simulink model "Quadcopter_State_model_Arduino"  (R2023b)
settings: Solver=VariableStepAuto  StartTime=0.0  StopTime=inf  FixedStep=0.00001  MinStep=0.001  RelTol=1e-3
model workspace (MAT data in the model file):
  DesiredPitchRoll : sugfis (value not decoded)
  DesiredThrust : sugfis (value not decoded)
  DesiredYaw : sugfis (value not decoded)
  Desired_Pitch = 0
  Desired_Roll = 0
  Desired_Yaw = 0
  Desired_Z_Velocity = -3
  FuzzyMotorspeed : sugfis (value not decoded)
values from neighbouring files (symbols this model uses):
  g = 9.81    [Quadcopter_Constants.m]
  Ixx = 0.0294838    [Quadcopter_Constants.m]
  Iyy = 0.0294838    [Quadcopter_Constants.m]
  Izz = 0.058967624    [Quadcopter_Constants.m]
  Jr = (6e-5)*1.358    (= 8.148e-05)    [Quadcopter_Constants.m]
  kd = 1    [Quadcopter_Constants.m]
  kd_phi = 1    [Quadcopter_Constants.m]
  kd_theta = 1    [Quadcopter_Constants.m]
  kf = 1    [Quadcopter_Constants.m]
  ki = 1    [Quadcopter_Constants.m]
  ki_phi = 1    [Quadcopter_Constants.m]
  ki_theta = 1    [Quadcopter_Constants.m]
  km = 4.74157e-9    (= 4.74157e-09)    [Quadcopter_Constants.m]
  kp = 1    [Quadcopter_Constants.m]
  kp_phi = 1    [Quadcopter_Constants.m]
  kp_theta = 1    [Quadcopter_Constants.m]
  kr = (0.1)*1.358    (= 0.1358)    [Quadcopter_Constants.m]
  kt = (0.1)*1.358    (= 0.1358)    [Quadcopter_Constants.m]
  l = 0.254    [Quadcopter_Constants.m]
  m = 0.914    [Quadcopter_Constants.m]
  sample_freq = 1000    [Quadcopter_Constants.m]
undefined symbols (not defined in the file or in its folder): LF
libraries: fuzblock x18, instrumentseriallib x12, simulink_extras x6, vrlib x4, instrumentlib x3, etargetslib x1, slpidlib x1, simulink x1
(part 2 of 5)

== system Quadcopter_State_model_Arduino/Arduino Sim/Control Panel ==
  note: Control Panel
  note: Enabling Results in
      | Simulation Lag
  Rocker Switch : RockerSwitchBlock
      settings: Values={{'Off', 'On'}, [0 1]}
  Rocker Switch1 : RockerSwitchBlock
      settings: Values={{'Off', 'On'}, [0 1]}
  Rocker Switch2 : RockerSwitchBlock
      settings: Values={{'Off', 'On'}, [0 1]}
  Rotary Switch : CustomTuningWebBlock  LabelPosition=Bottom  ShowInitialText=on  Configuration="{\"components\":[{\"name\":\"RotarySwitchComponent\",\"settings\":{\"arcAngle\":300,\"arcAngleOffset\":120,\"handle\":{\"size\":[150,150],\"src\":\"data:image\\/svg+xml;base64,PHN2ZyBpZD0iTGF5ZXJfMSIgZGF0YS1uYW1lPSJMYXllciAxIiB4bWxucz0iaHR0cDovL3d3dy53My5vcmcvMjAwMC9zdmciIHhtbG5zOnhsaW5rPSJodHRwOi8vd3d3LnczLm9yZy8xOTk5L3hsaW5rIiB2aWV3Qm94PSIwIDAgMTIxIDEyMSI+PGRlZnM+PHN0eWxlPi5jbHMtMXtmaWxsOnVybCgjbGluZWFyLWdyYWRpZW50KTt9LmNscy0yLC5jbHMtM3tmaWxsOiNkMWQxZDE7fS5jbHMtM3tzdHJva2U6I2I3YjdiNztzdHJva2UtbWl0ZXJsaW1pdDoxMDtzdHJva2Utd2lkdGg6MC4yNXB4O30uY2xzLTR7ZmlsbDojZjMwMDAwO30uY2xzLTV7ZmlsbDojZjIxNzY3O308L3N0eWxlPjxsaW5lYXJHcmFkaWVudCBpZD0ibGluZWFyLWdyYWRpZW50IiB4MT0iNjAuNSIgeTE9IjEyMC41IiB4Mj0iNjAuNSIgeTI9IjAuNSIgZ3JhZGllbnRVbml0cz0idXNlclNwYWNlT25Vc2UiPjxzdG9wIG9mZnNldD0iMCIgc3RvcC1jb2xvcj0iI2QxZDFkMSIvPjxzdG9wIG9mZnNldD0iMC4xIiBzdG9wLWNvbG9yPSIjY2VjZWNlIi8+PHN0b3Agb2Zmc2V0PSIwLjE5IiBzdG9wLWNvbG9yPSIjYzNjM2MzIi8+PHN0b3Agb2Zmc2V0PSIwLjI4IiBzdG9wLWNvbG9yPSIjYjFiMWIxIi8+PHN0b3Agb2Zmc2V0PSIwLjM2IiBzdG9wLWNvbG9yPSIjOTg5ODk4Ii8+PHN0b3Agb2Zmc2V0PSIwLjQ0IiBzdG9wLWNvbG9yPSIjNzg3ODc4Ii8+PHN0b3Agb2Zmc2V0PSIwLjQ2IiBzdG9wLWNvbG9yPSIjNmI2YjZiIi8+PHN0b3Agb2Zmc2V0PSIwLjU0IiBzdG9wLWNvbG9yPSIjNmI2YjZiIi8+PHN0b3Agb2Zmc2V0PSIwLjU2IiBzdG9wLWNvbG9yPSIjNzY3Njc2Ii8+PHN0b3Agb2Zmc2V0PSIwLjY0IiBzdG9wLWNvbG9yPSIjOTc5Nzk3Ii8+PHN0b3Agb2Zmc2V0PSIwLjcyIiBzdG9wLWNvbG9yPSIjYjBiMGIwIi8+PHN0b3Agb2Zmc2V0PSIwLjgxIiBzdG9wLWNvbG9yPSIjYzNjM2MzIi8+PHN0b3Agb2Zmc2V0PSIwLjkiIHN0b3AtY29sb3I9IiNjZGNkY2QiLz48c3RvcCBvZmZzZXQ9IjEiIHN0b3AtY29sb3I9IiNkMWQxZDEiLz48L2xpbmVhckdyYWRpZW50PjwvZGVmcz48Y2lyY2xlIGNsYXNzPSJjbHMtMSIgY3g9IjYwLjUiIGN5PSI2MC41IiByPSI2MCIvPjxwYXRoIGNsYXNzPSJjbHMtMiIgZD0iTTYwLjUsMUE1OS41LDU5LjUsMCwxLDEsMSw2MC41LDU5LjU3LDU5LjU3LDAsMCwxLDYwLjUsMW0wLTFBNjAuNSw2MC41LDAsMSwwLDEyMSw2MC41LDYwLjUsNjAuNSwwLDAsMCw2MC41LDBaIi8+PHJlY3QgY2xhc3M9ImNscy0zIiB4PSIwLjUiIHk9IjUxLjUiIHdpZHRoPSIxMjAiIGhlaWdodD0iMTgiIHJ4PSIzLjA0Ii8+PHJlY3QgY2xhc3M9ImNscy00IiB4PSI1Ljc1IiB5PSI1OC43NSIgd2lkdGg9IjE2IiBoZWlnaHQ9IjMiLz48cGF0aCBjbGFzcz0iY2xzLTUiIGQ9Ik0yMS4yNSw1OS4yNXYyaC0xNXYtMmgxNW0xLTFoLTE3djRoMTd2LTRaIi8+PC9zdmc+\"},\"handleOffset\":[0,0],\"handleOrientation\":180,\"handlePosition\":[0,0,1,1],\"handleSize\":{\"height\":0.5,\"width\":0.5},\"labelRadius\":0.36,\"position\":[0,0,1,1],\"states\":[{\"Label\":{\"color\":[0,0,0,1],\"icon\":{\"size\":[0,0],\"src\":[],\"srcOrientation\":\"Right\"},\"iconPlacement\":\"left\",\"opacity\":1,\"position\":[0.7345552884615385,0.6796274038461538],\"show\":true,\"text\":{\"content\":\"-128\",\"font\":\"Helvetica\",\"fontSize\":24}},\"Value\":-128},{\"Label\":{\"color\":[0,0,0,1],\"icon\":{\"size\":[0,0],\"src\":[],\"srcOrientation\":\"Right\"},\"iconPlacement\":\"left\",\"opacity\":1,\"position\":[0.36532451923076925,0.1180889423076923],\"show\":true,\"text\":{\"content\":\"-97\",\"font\":\"Helvetica\",\"fontSize\":24}},\"Value\":-97},{\"Label\":{\"color\":[0,0,0,1],\"icon\":{\"size\":[0,0],\"src\":[],\"srcOrientation\":\"Right\"},\"iconPlacement\":\"left\",\"opacity\":1,\"position\":[0.7191706730769231,0.19501201923076922],\"show\":true,\"text\":{\"content\":\"-65\",\"font\":\"Helvetica\",\"fontSize\":24}},\"Value\":-65},{\"Label\":{\"color\":[0,0,0,1],\"icon\":{\"size\":[0,0],\"src\":[],\"srcOrientation\":\"Right\"},\"iconPlacement\":\"left\",\"opacity\":1,\"position\":[0.35757211538461536,0.7603966346153846],\"show\":true,\"text\":{\"content\":\"-33\",\"font\":\"Helvetica\",\"fontSize\":24}},\"Value\":-33},{\"Label\":{\"color\":[0,0,0,1],\"icon\":{\"size\":[0,0],\"src\":[],\"srcOrientation\":\"Right\"},\"iconPlacement\":\"left\",\"opacity\":1,\"position\":[0.09603365384615385,0.46033653846153844],\"show\":true,\"text\":{\"content\":\"0\",\"font\":\"Helvetica\",\"fontSize\":24}},\"Value\":0},{\"Label\":{\"color\":[0,0,0,1],\"icon\":{\"size\":[0,0],\"src\":[],\"srcOrientation\":\"Right\"},\"iconPlacement\":\"left\",\"opacity\":1,\"position\":[0.7191706730769231,0.19501201923076922],\"show\":true,\"text\":{\"content\":\"32\",\"font\":\"Helvetica\",\"fontSize\":24}},\"Value\":32},{\"Label\":{\"color\":[0,0,0,1],\"icon\":{\"size\":[0,0],\"src\":[],\"srcOrientation\":\"Right\"},\"iconPlacement\":\"left\",\"opacity\":1,\"position\":[0.7191706730769231,0.19501201923076922],\"show\":true,\"text\":{\"content\":\"64\",\"font\":\"Helvetica\",\"fontSize\":24}},\"Value\":64},{\"Label\":{\"color\":[0,0,0,1],\"icon\":{\"size\":[0,0],\"src\":[],\"srcOrientation\":\"Right\"},\"iconPlacement\":\"left\",\"opacity\":1,\"position\":[0.7191706730769231,0.19501201923076922],\"show\":true,\"text\":{\"content\":\"96\",\"font\":\"Helvetica\",\"fontSize\":24}},\"Value\":96},{\"Label\":{\"color\":[0,0,0,1],\"icon\":{\"size\":[0,0],\"src\":[],\"srcOrientation\":\"Right\"},\"iconPlacement\":\"left\",\"opacity\":1,\"position\":[0.7191706730769231,0.19501201923076922],\"show\":true,\"text\":{\"content\":\"127\",\"font\":\"Helvetica\",\"fontSize\":24}},\"Value\":127}],\"tickRadius\":0.32}},{\"name\":\"BackgroundImageComponent\",\"settings\":{\"image\":{\"size\":[155,150],\"src\":\"data:image\\/svg+xml;base64,PD94bWwgdmVyc2lvbj0iMS4wIiBlbmNvZGluZz0idXRmLTgiPz4NCjwhLS0gR2VuZXJhdG9yOiBBZG9iZSBJbGx1c3RyYXRvciAyNS4wLjAsIFNWRyBFeHBvcnQgUGx1Zy1JbiAuIFNWRyBWZXJzaW9uOiA2LjAwIEJ1aWxkIDApICAtLT4NCjxzdmcgdmVyc2lvbj0iMS4xIg0KCSBpZD0iTGF5ZXJfMl8xXyIgeG1sbnM6Y2M9Imh0dHA6Ly9jcmVhdGl2ZWNvbW1vbnMub3JnL25zIyIgeG1sbnM6ZGM9Imh0dHA6Ly9wdXJsLm9yZy9kYy9lbGVtZW50cy8xLjEvIiB4bWxuczppbmtzY2FwZT0iaHR0cDovL3d3dy5pbmtzY2FwZS5vcmcv ...(+4184 chars)\",\"srcOrientation\":\"Right\"},\"position\":[0,0,1,1],\"scaleMode\":\"0\"}},{\"name\":\"ForegroundImageComponent\",\"settings\":{\"image\":{\"size\":[0,0],\"src\":\"default\",\"srcOrientation\":[]},\"isForeground\":1,\"position\":[0,0,1,1],\"scaleMode\":\"0\"}}],\"settings\":{\"BindingType\":\"param\",\"backgroundColor\":[0,0,255,\"1\"],\"backgroundOffset\":1,\"fixedAspectRatio\":\"on\",\"image\":{\"size\":[150,150],\"src\":\"data:image\\/svg+xml;base64,PD94bWwgdmVyc2lvbj0iMS4wIiBlbmNvZGluZz0iVVRGLTgiIHN0YW5kYWxvbmU9Im5vIj8+CjwhLS0gR2VuZXJhdG9yOiBBZG9iZSBJbGx1c3RyYXRvciAxOS4yLjEsIFNWRyBFeHBvcnQgUGx1Zy1JbiAuIFNWRyBWZXJzaW9uOiA2LjAwIEJ1aWxkIDApICAtLT4KCjxzdmcKICAgeG1sbnM6ZGM9Imh0dHA6Ly9wdXJsLm9yZy9kYy9lbGVtZW50cy8xLjEvIgogICB4bWxuczpjYz0iaHR0cDovL2NyZWF0aXZlY29tbW9ucy5vcmcvbnMjIgogICB4bWxuczpyZGY9Imh0dHA6Ly93d3cudzMub3JnLzE5OTkvMDIvMjItcmRmLXN5bnRh ...(+9660 chars)\"},\"showBackgroundColor\":false,\"variant\":\"rotarySwitch\",\"version\":\"R2022b\"},\"type\":\"RotarySwitch\"}"
  Rotary Switch1 : CustomTuningWebBlock  LabelPosition=Bottom  ShowInitialText=on  Configuration="{\"components\":[{\"name\":\"RotarySwitchComponent\",\"settings\":{\"arcAngle\":300,\"arcAngleOffset\":120,\"handle\":{\"size\":[150,150],\"src\":\"data:image\\/svg+xml;base64,PHN2ZyBpZD0iTGF5ZXJfMSIgZGF0YS1uYW1lPSJMYXllciAxIiB4bWxucz0iaHR0cDovL3d3dy53My5vcmcvMjAwMC9zdmciIHhtbG5zOnhsaW5rPSJodHRwOi8vd3d3LnczLm9yZy8xOTk5L3hsaW5rIiB2aWV3Qm94PSIwIDAgMTIxIDEyMSI+PGRlZnM+PHN0eWxlPi5jbHMtMXtmaWxsOnVybCgjbGluZWFyLWdyYWRpZW50KTt9LmNscy0yLC5jbHMtM3tmaWxsOiNkMWQxZDE7fS5jbHMtM3tzdHJva2U6I2I3YjdiNztzdHJva2UtbWl0ZXJsaW1pdDoxMDtzdHJva2Utd2lkdGg6MC4yNXB4O30uY2xzLTR7ZmlsbDojZjMwMDAwO30uY2xzLTV7ZmlsbDojZjIxNzY3O308L3N0eWxlPjxsaW5lYXJHcmFkaWVudCBpZD0ibGluZWFyLWdyYWRpZW50IiB4MT0iNjAuNSIgeTE9IjEyMC41IiB4Mj0iNjAuNSIgeTI9IjAuNSIgZ3JhZGllbnRVbml0cz0idXNlclNwYWNlT25Vc2UiPjxzdG9wIG9mZnNldD0iMCIgc3RvcC1jb2xvcj0iI2QxZDFkMSIvPjxzdG9wIG9mZnNldD0iMC4xIiBzdG9wLWNvbG9yPSIjY2VjZWNlIi8+PHN0b3Agb2Zmc2V0PSIwLjE5IiBzdG9wLWNvbG9yPSIjYzNjM2MzIi8+PHN0b3Agb2Zmc2V0PSIwLjI4IiBzdG9wLWNvbG9yPSIjYjFiMWIxIi8+PHN0b3Agb2Zmc2V0PSIwLjM2IiBzdG9wLWNvbG9yPSIjOTg5ODk4Ii8+PHN0b3Agb2Zmc2V0PSIwLjQ0IiBzdG9wLWNvbG9yPSIjNzg3ODc4Ii8+PHN0b3Agb2Zmc2V0PSIwLjQ2IiBzdG9wLWNvbG9yPSIjNmI2YjZiIi8+PHN0b3Agb2Zmc2V0PSIwLjU0IiBzdG9wLWNvbG9yPSIjNmI2YjZiIi8+PHN0b3Agb2Zmc2V0PSIwLjU2IiBzdG9wLWNvbG9yPSIjNzY3Njc2Ii8+PHN0b3Agb2Zmc2V0PSIwLjY0IiBzdG9wLWNvbG9yPSIjOTc5Nzk3Ii8+PHN0b3Agb2Zmc2V0PSIwLjcyIiBzdG9wLWNvbG9yPSIjYjBiMGIwIi8+PHN0b3Agb2Zmc2V0PSIwLjgxIiBzdG9wLWNvbG9yPSIjYzNjM2MzIi8+PHN0b3Agb2Zmc2V0PSIwLjkiIHN0b3AtY29sb3I9IiNjZGNkY2QiLz48c3RvcCBvZmZzZXQ9IjEiIHN0b3AtY29sb3I9IiNkMWQxZDEiLz48L2xpbmVhckdyYWRpZW50PjwvZGVmcz48Y2lyY2xlIGNsYXNzPSJjbHMtMSIgY3g9IjYwLjUiIGN5PSI2MC41IiByPSI2MCIvPjxwYXRoIGNsYXNzPSJjbHMtMiIgZD0iTTYwLjUsMUE1OS41LDU5LjUsMCwxLDEsMSw2MC41LDU5LjU3LDU5LjU3LDAsMCwxLDYwLjUsMW0wLTFBNjAuNSw2MC41LDAsMSwwLDEyMSw2MC41LDYwLjUsNjAuNSwwLDAsMCw2MC41LDBaIi8+PHJlY3QgY2xhc3M9ImNscy0zIiB4PSIwLjUiIHk9IjUxLjUiIHdpZHRoPSIxMjAiIGhlaWdodD0iMTgiIHJ4PSIzLjA0Ii8+PHJlY3QgY2xhc3M9ImNscy00IiB4PSI1Ljc1IiB5PSI1OC43NSIgd2lkdGg9IjE2IiBoZWlnaHQ9IjMiLz48cGF0aCBjbGFzcz0iY2xzLTUiIGQ9Ik0yMS4yNSw1OS4yNXYyaC0xNXYtMmgxNW0xLTFoLTE3djRoMTd2LTRaIi8+PC9zdmc+\"},\"handleOffset\":[0,0],\"handleOrientation\":180,\"handlePosition\":[0,0,1,1],\"handleSize\":{\"height\":0.5,\"width\":0.5},\"labelRadius\":0.36,\"position\":[0,0,1,1],\"states\":[{\"Label\":{\"color\":[0,0,0,1],\"icon\":{\"size\":[0,0],\"src\":[],\"srcOrientation\":\"Right\"},\"iconPlacement\":\"left\",\"opacity\":1,\"position\":[0.7345552884615385,0.6796274038461538],\"show\":true,\"text\":{\"content\":\"-127\",\"font\":\"Helvetica\",\"fontSize\":24}},\"Value\":-127},{\"Label\":{\"color\":[0,0,0,1],\"icon\":{\"size\":[0,0],\"src\":[],\"srcOrientation\":\"Right\"},\"iconPlacement\":\"left\",\"opacity\":1,\"position\":[0.36532451923076925,0.1180889423076923],\"show\":true,\"text\":{\"content\":\"-96\",\"font\":\"Helvetica\",\"fontSize\":24}},\"Value\":-96},{\"Label\":{\"color\":[0,0,0,1],\"icon\":{\"size\":[0,0],\"src\":[],\"srcOrientation\":\"Right\"},\"iconPlacement\":\"left\",\"opacity\":1,\"position\":[0.7191706730769231,0.19501201923076922],\"show\":true,\"text\":{\"content\":\"-64\",\"font\":\"Helvetica\",\"fontSize\":24}},\"Value\":-64},{\"Label\":{\"color\":[0,0,0,1],\"icon\":{\"size\":[0,0],\"src\":[],\"srcOrientation\":\"Right\"},\"iconPlacement\":\"left\",\"opacity\":1,\"position\":[0.35757211538461536,0.7603966346153846],\"show\":true,\"text\":{\"content\":\"-32\",\"font\":\"Helvetica\",\"fontSize\":24}},\"Value\":-32},{\"Label\":{\"color\":[0,0,0,1],\"icon\":{\"size\":[0,0],\"src\":[],\"srcOrientation\":\"Right\"},\"iconPlacement\":\"left\",\"opacity\":1,\"position\":[0.09603365384615385,0.46033653846153844],\"show\":true,\"text\":{\"content\":\"0\",\"font\":\"Helvetica\",\"fontSize\":24}},\"Value\":0},{\"Label\":{\"color\":[0,0,0,1],\"icon\":{\"size\":[0,0],\"src\":[],\"srcOrientation\":\"Right\"},\"iconPlacement\":\"left\",\"opacity\":1,\"position\":[0.7191706730769231,0.19501201923076922],\"show\":true,\"text\":{\"content\":\"32\",\"font\":\"Helvetica\",\"fontSize\":24}},\"Value\":32},{\"Label\":{\"color\":[0,0,0,1],\"icon\":{\"size\":[0,0],\"src\":[],\"srcOrientation\":\"Right\"},\"iconPlacement\":\"left\",\"opacity\":1,\"position\":[0.7191706730769231,0.19501201923076922],\"show\":true,\"text\":{\"content\":\"64\",\"font\":\"Helvetica\",\"fontSize\":24}},\"Value\":64},{\"Label\":{\"color\":[0,0,0,1],\"icon\":{\"size\":[0,0],\"src\":[],\"srcOrientation\":\"Right\"},\"iconPlacement\":\"left\",\"opacity\":1,\"position\":[0.7191706730769231,0.19501201923076922],\"show\":true,\"text\":{\"content\":\"96\",\"font\":\"Helvetica\",\"fontSize\":24}},\"Value\":96},{\"Label\":{\"color\":[0,0,0,1],\"icon\":{\"size\":[0,0],\"src\":[],\"srcOrientation\":\"Right\"},\"iconPlacement\":\"left\",\"opacity\":1,\"position\":[0.7191706730769231,0.19501201923076922],\"show\":true,\"text\":{\"content\":\"127\",\"font\":\"Helvetica\",\"fontSize\":24}},\"Value\":127}],\"tickRadius\":0.32}},{\"name\":\"BackgroundImageComponent\",\"settings\":{\"image\":{\"size\":[155,150],\"src\":\"data:image\\/svg+xml;base64,PD94bWwgdmVyc2lvbj0iMS4wIiBlbmNvZGluZz0idXRmLTgiPz4NCjwhLS0gR2VuZXJhdG9yOiBBZG9iZSBJbGx1c3RyYXRvciAyNS4wLjAsIFNWRyBFeHBvcnQgUGx1Zy1JbiAuIFNWRyBWZXJzaW9uOiA2LjAwIEJ1aWxkIDApICAtLT4NCjxzdmcgdmVyc2lvbj0iMS4xIg0KCSBpZD0iTGF5ZXJfMl8xXyIgeG1sbnM6Y2M9Imh0dHA6Ly9jcmVhdGl2ZWNvbW1vbnMub3JnL25zIyIgeG1sbnM6ZGM9Imh0dHA6Ly9wdXJsLm9yZy9kYy9lbGVtZW50cy8xLjEvIiB4bWxuczppbmtzY2FwZT0iaHR0cDovL3d3dy5pbmtzY2FwZS5vcmcv ...(+4184 chars)\",\"srcOrientation\":\"Right\"},\"position\":[0,0,1,1],\"scaleMode\":\"0\"}},{\"name\":\"ForegroundImageComponent\",\"settings\":{\"image\":{\"size\":[0,0],\"src\":\"default\",\"srcOrientation\":[]},\"isForeground\":1,\"position\":[0,0,1,1],\"scaleMode\":\"0\"}}],\"settings\":{\"BindingType\":\"param\",\"backgroundColor\":[0,0,255,\"1\"],\"backgroundOffset\":1,\"fixedAspectRatio\":\"on\",\"image\":{\"size\":[150,150],\"src\":\"data:image\\/svg+xml;base64,PD94bWwgdmVyc2lvbj0iMS4wIiBlbmNvZGluZz0iVVRGLTgiIHN0YW5kYWxvbmU9Im5vIj8+CjwhLS0gR2VuZXJhdG9yOiBBZG9iZSBJbGx1c3RyYXRvciAxOS4yLjEsIFNWRyBFeHBvcnQgUGx1Zy1JbiAuIFNWRyBWZXJzaW9uOiA2LjAwIEJ1aWxkIDApICAtLT4KCjxzdmcKICAgeG1sbnM6ZGM9Imh0dHA6Ly9wdXJsLm9yZy9kYy9lbGVtZW50cy8xLjEvIgogICB4bWxuczpjYz0iaHR0cDovL2NyZWF0aXZlY29tbW9ucy5vcmcvbnMjIgogICB4bWxuczpyZGY9Imh0dHA6Ly93d3cudzMub3JnLzE5OTkvMDIvMjItcmRmLXN5bnRh ...(+9660 chars)\"},\"showBackgroundColor\":false,\"variant\":\"rotarySwitch\",\"version\":\"R2022b\"},\"type\":\"RotarySwitch\"}"
  Rotary Switch2 : CustomTuningWebBlock  LabelPosition=Bottom  ShowInitialText=on  Configuration="{\"components\":[{\"name\":\"RotarySwitchComponent\",\"settings\":{\"arcAngle\":300,\"arcAngleOffset\":120,\"handle\":{\"size\":[150,150],\"src\":\"data:image\\/svg+xml;base64,PHN2ZyBpZD0iTGF5ZXJfMSIgZGF0YS1uYW1lPSJMYXllciAxIiB4bWxucz0iaHR0cDovL3d3dy53My5vcmcvMjAwMC9zdmciIHhtbG5zOnhsaW5rPSJodHRwOi8vd3d3LnczLm9yZy8xOTk5L3hsaW5rIiB2aWV3Qm94PSIwIDAgMTIxIDEyMSI+PGRlZnM+PHN0eWxlPi5jbHMtMXtmaWxsOnVybCgjbGluZWFyLWdyYWRpZW50KTt9LmNscy0yLC5jbHMtM3tmaWxsOiNkMWQxZDE7fS5jbHMtM3tzdHJva2U6I2I3YjdiNztzdHJva2UtbWl0ZXJsaW1pdDoxMDtzdHJva2Utd2lkdGg6MC4yNXB4O30uY2xzLTR7ZmlsbDojZjMwMDAwO30uY2xzLTV7ZmlsbDojZjIxNzY3O308L3N0eWxlPjxsaW5lYXJHcmFkaWVudCBpZD0ibGluZWFyLWdyYWRpZW50IiB4MT0iNjAuNSIgeTE9IjEyMC41IiB4Mj0iNjAuNSIgeTI9IjAuNSIgZ3JhZGllbnRVbml0cz0idXNlclNwYWNlT25Vc2UiPjxzdG9wIG9mZnNldD0iMCIgc3RvcC1jb2xvcj0iI2QxZDFkMSIvPjxzdG9wIG9mZnNldD0iMC4xIiBzdG9wLWNvbG9yPSIjY2VjZWNlIi8+PHN0b3Agb2Zmc2V0PSIwLjE5IiBzdG9wLWNvbG9yPSIjYzNjM2MzIi8+PHN0b3Agb2Zmc2V0PSIwLjI4IiBzdG9wLWNvbG9yPSIjYjFiMWIxIi8+PHN0b3Agb2Zmc2V0PSIwLjM2IiBzdG9wLWNvbG9yPSIjOTg5ODk4Ii8+PHN0b3Agb2Zmc2V0PSIwLjQ0IiBzdG9wLWNvbG9yPSIjNzg3ODc4Ii8+PHN0b3Agb2Zmc2V0PSIwLjQ2IiBzdG9wLWNvbG9yPSIjNmI2YjZiIi8+PHN0b3Agb2Zmc2V0PSIwLjU0IiBzdG9wLWNvbG9yPSIjNmI2YjZiIi8+PHN0b3Agb2Zmc2V0PSIwLjU2IiBzdG9wLWNvbG9yPSIjNzY3Njc2Ii8+PHN0b3Agb2Zmc2V0PSIwLjY0IiBzdG9wLWNvbG9yPSIjOTc5Nzk3Ii8+PHN0b3Agb2Zmc2V0PSIwLjcyIiBzdG9wLWNvbG9yPSIjYjBiMGIwIi8+PHN0b3Agb2Zmc2V0PSIwLjgxIiBzdG9wLWNvbG9yPSIjYzNjM2MzIi8+PHN0b3Agb2Zmc2V0PSIwLjkiIHN0b3AtY29sb3I9IiNjZGNkY2QiLz48c3RvcCBvZmZzZXQ9IjEiIHN0b3AtY29sb3I9IiNkMWQxZDEiLz48L2xpbmVhckdyYWRpZW50PjwvZGVmcz48Y2lyY2xlIGNsYXNzPSJjbHMtMSIgY3g9IjYwLjUiIGN5PSI2MC41IiByPSI2MCIvPjxwYXRoIGNsYXNzPSJjbHMtMiIgZD0iTTYwLjUsMUE1OS41LDU5LjUsMCwxLDEsMSw2MC41LDU5LjU3LDU5LjU3LDAsMCwxLDYwLjUsMW0wLTFBNjAuNSw2MC41LDAsMSwwLDEyMSw2MC41LDYwLjUsNjAuNSwwLDAsMCw2MC41LDBaIi8+PHJlY3QgY2xhc3M9ImNscy0zIiB4PSIwLjUiIHk9IjUxLjUiIHdpZHRoPSIxMjAiIGhlaWdodD0iMTgiIHJ4PSIzLjA0Ii8+PHJlY3QgY2xhc3M9ImNscy00IiB4PSI1Ljc1IiB5PSI1OC43NSIgd2lkdGg9IjE2IiBoZWlnaHQ9IjMiLz48cGF0aCBjbGFzcz0iY2xzLTUiIGQ9Ik0yMS4yNSw1OS4yNXYyaC0xNXYtMmgxNW0xLTFoLTE3djRoMTd2LTRaIi8+PC9zdmc+\"},\"handleOffset\":[0,0],\"handleOrientation\":180,\"handlePosition\":[0,0,1,1],\"handleSize\":{\"height\":0.5,\"width\":0.5},\"labelRadius\":0.36,\"position\":[0,0,1,1],\"states\":[{\"Label\":{\"color\":[0,0,0,1],\"icon\":{\"size\":[0,0],\"src\":[],\"srcOrientation\":\"Right\"},\"iconPlacement\":\"left\",\"opacity\":1,\"position\":[0.7345552884615385,0.6796274038461538],\"show\":true,\"text\":{\"content\":\"-127\",\"font\":\"Helvetica\",\"fontSize\":24}},\"Value\":-127},{\"Label\":{\"color\":[0,0,0,1],\"icon\":{\"size\":[0,0],\"src\":[],\"srcOrientation\":\"Right\"},\"iconPlacement\":\"left\",\"opacity\":1,\"position\":[0.36532451923076925,0.1180889423076923],\"show\":true,\"text\":{\"content\":\"-96\",\"font\":\"Helvetica\",\"fontSize\":24}},\"Value\":-96},{\"Label\":{\"color\":[0,0,0,1],\"icon\":{\"size\":[0,0],\"src\":[],\"srcOrientation\":\"Right\"},\"iconPlacement\":\"left\",\"opacity\":1,\"position\":[0.7191706730769231,0.19501201923076922],\"show\":true,\"text\":{\"content\":\"-64\",\"font\":\"Helvetica\",\"fontSize\":24}},\"Value\":-64},{\"Label\":{\"color\":[0,0,0,1],\"icon\":{\"size\":[0,0],\"src\":[],\"srcOrientation\":\"Right\"},\"iconPlacement\":\"left\",\"opacity\":1,\"position\":[0.35757211538461536,0.7603966346153846],\"show\":true,\"text\":{\"content\":\"-32\",\"font\":\"Helvetica\",\"fontSize\":24}},\"Value\":-32},{\"Label\":{\"color\":[0,0,0,1],\"icon\":{\"size\":[0,0],\"src\":[],\"srcOrientation\":\"Right\"},\"iconPlacement\":\"left\",\"opacity\":1,\"position\":[0.09603365384615385,0.46033653846153844],\"show\":true,\"text\":{\"content\":\"0\",\"font\":\"Helvetica\",\"fontSize\":24}},\"Value\":0},{\"Label\":{\"color\":[0,0,0,1],\"icon\":{\"size\":[0,0],\"src\":[],\"srcOrientation\":\"Right\"},\"iconPlacement\":\"left\",\"opacity\":1,\"position\":[0.7191706730769231,0.19501201923076922],\"show\":true,\"text\":{\"content\":\"32\",\"font\":\"Helvetica\",\"fontSize\":24}},\"Value\":32},{\"Label\":{\"color\":[0,0,0,1],\"icon\":{\"size\":[0,0],\"src\":[],\"srcOrientation\":\"Right\"},\"iconPlacement\":\"left\",\"opacity\":1,\"position\":[0.7191706730769231,0.19501201923076922],\"show\":true,\"text\":{\"content\":\"64\",\"font\":\"Helvetica\",\"fontSize\":24}},\"Value\":64},{\"Label\":{\"color\":[0,0,0,1],\"icon\":{\"size\":[0,0],\"src\":[],\"srcOrientation\":\"Right\"},\"iconPlacement\":\"left\",\"opacity\":1,\"position\":[0.7191706730769231,0.19501201923076922],\"show\":true,\"text\":{\"content\":\"96\",\"font\":\"Helvetica\",\"fontSize\":24}},\"Value\":96},{\"Label\":{\"color\":[0,0,0,1],\"icon\":{\"size\":[0,0],\"src\":[],\"srcOrientation\":\"Right\"},\"iconPlacement\":\"left\",\"opacity\":1,\"position\":[0.7191706730769231,0.19501201923076922],\"show\":true,\"text\":{\"content\":\"127\",\"font\":\"Helvetica\",\"fontSize\":24}},\"Value\":127}],\"tickRadius\":0.32}},{\"name\":\"BackgroundImageComponent\",\"settings\":{\"image\":{\"size\":[155,150],\"src\":\"data:image\\/svg+xml;base64,PD94bWwgdmVyc2lvbj0iMS4wIiBlbmNvZGluZz0idXRmLTgiPz4NCjwhLS0gR2VuZXJhdG9yOiBBZG9iZSBJbGx1c3RyYXRvciAyNS4wLjAsIFNWRyBFeHBvcnQgUGx1Zy1JbiAuIFNWRyBWZXJzaW9uOiA2LjAwIEJ1aWxkIDApICAtLT4NCjxzdmcgdmVyc2lvbj0iMS4xIg0KCSBpZD0iTGF5ZXJfMl8xXyIgeG1sbnM6Y2M9Imh0dHA6Ly9jcmVhdGl2ZWNvbW1vbnMub3JnL25zIyIgeG1sbnM6ZGM9Imh0dHA6Ly9wdXJsLm9yZy9kYy9lbGVtZW50cy8xLjEvIiB4bWxuczppbmtzY2FwZT0iaHR0cDovL3d3dy5pbmtzY2FwZS5vcmcv ...(+4184 chars)\",\"srcOrientation\":\"Right\"},\"position\":[0,0,1,1],\"scaleMode\":\"0\"}},{\"name\":\"ForegroundImageComponent\",\"settings\":{\"image\":{\"size\":[0,0],\"src\":\"default\",\"srcOrientation\":[]},\"isForeground\":1,\"position\":[0,0,1,1],\"scaleMode\":\"0\"}}],\"settings\":{\"BindingType\":\"param\",\"backgroundColor\":[0,0,255,\"1\"],\"backgroundOffset\":1,\"fixedAspectRatio\":\"on\",\"image\":{\"size\":[150,150],\"src\":\"data:image\\/svg+xml;base64,PD94bWwgdmVyc2lvbj0iMS4wIiBlbmNvZGluZz0iVVRGLTgiIHN0YW5kYWxvbmU9Im5vIj8+CjwhLS0gR2VuZXJhdG9yOiBBZG9iZSBJbGx1c3RyYXRvciAxOS4yLjEsIFNWRyBFeHBvcnQgUGx1Zy1JbiAuIFNWRyBWZXJzaW9uOiA2LjAwIEJ1aWxkIDApICAtLT4KCjxzdmcKICAgeG1sbnM6ZGM9Imh0dHA6Ly9wdXJsLm9yZy9kYy9lbGVtZW50cy8xLjEvIgogICB4bWxuczpjYz0iaHR0cDovL2NyZWF0aXZlY29tbW9ucy5vcmcvbnMjIgogICB4bWxuczpyZGY9Imh0dHA6Ly93d3cudzMub3JnLzE5OTkvMDIvMjItcmRmLXN5bnRh ...(+9660 chars)\"},\"showBackgroundColor\":false,\"variant\":\"rotarySwitch\",\"version\":\"R2022b\"},\"type\":\"RotarySwitch\"}"
  Rotary Switch3 : CustomTuningWebBlock  LabelPosition=Bottom  ShowInitialText=on  Configuration="{\"components\":[{\"name\":\"RotarySwitchComponent\",\"settings\":{\"arcAngle\":300,\"arcAngleOffset\":120,\"handle\":{\"size\":[150,150],\"src\":\"data:image\\/svg+xml;base64,PHN2ZyBpZD0iTGF5ZXJfMSIgZGF0YS1uYW1lPSJMYXllciAxIiB4bWxucz0iaHR0cDovL3d3dy53My5vcmcvMjAwMC9zdmciIHhtbG5zOnhsaW5rPSJodHRwOi8vd3d3LnczLm9yZy8xOTk5L3hsaW5rIiB2aWV3Qm94PSIwIDAgMTIxIDEyMSI+PGRlZnM+PHN0eWxlPi5jbHMtMXtmaWxsOnVybCgjbGluZWFyLWdyYWRpZW50KTt9LmNscy0yLC5jbHMtM3tmaWxsOiNkMWQxZDE7fS5jbHMtM3tzdHJva2U6I2I3YjdiNztzdHJva2UtbWl0ZXJsaW1pdDoxMDtzdHJva2Utd2lkdGg6MC4yNXB4O30uY2xzLTR7ZmlsbDojZjMwMDAwO30uY2xzLTV7ZmlsbDojZjIxNzY3O308L3N0eWxlPjxsaW5lYXJHcmFkaWVudCBpZD0ibGluZWFyLWdyYWRpZW50IiB4MT0iNjAuNSIgeTE9IjEyMC41IiB4Mj0iNjAuNSIgeTI9IjAuNSIgZ3JhZGllbnRVbml0cz0idXNlclNwYWNlT25Vc2UiPjxzdG9wIG9mZnNldD0iMCIgc3RvcC1jb2xvcj0iI2QxZDFkMSIvPjxzdG9wIG9mZnNldD0iMC4xIiBzdG9wLWNvbG9yPSIjY2VjZWNlIi8+PHN0b3Agb2Zmc2V0PSIwLjE5IiBzdG9wLWNvbG9yPSIjYzNjM2MzIi8+PHN0b3Agb2Zmc2V0PSIwLjI4IiBzdG9wLWNvbG9yPSIjYjFiMWIxIi8+PHN0b3Agb2Zmc2V0PSIwLjM2IiBzdG9wLWNvbG9yPSIjOTg5ODk4Ii8+PHN0b3Agb2Zmc2V0PSIwLjQ0IiBzdG9wLWNvbG9yPSIjNzg3ODc4Ii8+PHN0b3Agb2Zmc2V0PSIwLjQ2IiBzdG9wLWNvbG9yPSIjNmI2YjZiIi8+PHN0b3Agb2Zmc2V0PSIwLjU0IiBzdG9wLWNvbG9yPSIjNmI2YjZiIi8+PHN0b3Agb2Zmc2V0PSIwLjU2IiBzdG9wLWNvbG9yPSIjNzY3Njc2Ii8+PHN0b3Agb2Zmc2V0PSIwLjY0IiBzdG9wLWNvbG9yPSIjOTc5Nzk3Ii8+PHN0b3Agb2Zmc2V0PSIwLjcyIiBzdG9wLWNvbG9yPSIjYjBiMGIwIi8+PHN0b3Agb2Zmc2V0PSIwLjgxIiBzdG9wLWNvbG9yPSIjYzNjM2MzIi8+PHN0b3Agb2Zmc2V0PSIwLjkiIHN0b3AtY29sb3I9IiNjZGNkY2QiLz48c3RvcCBvZmZzZXQ9IjEiIHN0b3AtY29sb3I9IiNkMWQxZDEiLz48L2xpbmVhckdyYWRpZW50PjwvZGVmcz48Y2lyY2xlIGNsYXNzPSJjbHMtMSIgY3g9IjYwLjUiIGN5PSI2MC41IiByPSI2MCIvPjxwYXRoIGNsYXNzPSJjbHMtMiIgZD0iTTYwLjUsMUE1OS41LDU5LjUsMCwxLDEsMSw2MC41LDU5LjU3LDU5LjU3LDAsMCwxLDYwLjUsMW0wLTFBNjAuNSw2MC41LDAsMSwwLDEyMSw2MC41LDYwLjUsNjAuNSwwLDAsMCw2MC41LDBaIi8+PHJlY3QgY2xhc3M9ImNscy0zIiB4PSIwLjUiIHk9IjUxLjUiIHdpZHRoPSIxMjAiIGhlaWdodD0iMTgiIHJ4PSIzLjA0Ii8+PHJlY3QgY2xhc3M9ImNscy00IiB4PSI1Ljc1IiB5PSI1OC43NSIgd2lkdGg9IjE2IiBoZWlnaHQ9IjMiLz48cGF0aCBjbGFzcz0iY2xzLTUiIGQ9Ik0yMS4yNSw1OS4yNXYyaC0xNXYtMmgxNW0xLTFoLTE3djRoMTd2LTRaIi8+PC9zdmc+\"},\"handleOffset\":[0,0],\"handleOrientation\":180,\"handlePosition\":[0,0,1,1],\"handleSize\":{\"height\":0.5,\"width\":0.5},\"labelRadius\":0.36,\"position\":[0,0,1,1],\"states\":[{\"Label\":{\"color\":[0,0,0,1],\"icon\":{\"size\":[0,0],\"src\":[],\"srcOrientation\":\"Right\"},\"iconPlacement\":\"left\",\"opacity\":1,\"position\":[0.7345552884615385,0.6796274038461538],\"show\":true,\"text\":{\"content\":\"-127\",\"font\":\"Helvetica\",\"fontSize\":24}},\"Value\":-127},{\"Label\":{\"color\":[0,0,0,1],\"icon\":{\"size\":[0,0],\"src\":[],\"srcOrientation\":\"Right\"},\"iconPlacement\":\"left\",\"opacity\":1,\"position\":[0.36532451923076925,0.1180889423076923],\"show\":true,\"text\":{\"content\":\"-96\",\"font\":\"Helvetica\",\"fontSize\":24}},\"Value\":-96},{\"Label\":{\"color\":[0,0,0,1],\"icon\":{\"size\":[0,0],\"src\":[],\"srcOrientation\":\"Right\"},\"iconPlacement\":\"left\",\"opacity\":1,\"position\":[0.7191706730769231,0.19501201923076922],\"show\":true,\"text\":{\"content\":\"-64\",\"font\":\"Helvetica\",\"fontSize\":24}},\"Value\":-64},{\"Label\":{\"color\":[0,0,0,1],\"icon\":{\"size\":[0,0],\"src\":[],\"srcOrientation\":\"Right\"},\"iconPlacement\":\"left\",\"opacity\":1,\"position\":[0.35757211538461536,0.7603966346153846],\"show\":true,\"text\":{\"content\":\"-32\",\"font\":\"Helvetica\",\"fontSize\":24}},\"Value\":-32},{\"Label\":{\"color\":[0,0,0,1],\"icon\":{\"size\":[0,0],\"src\":[],\"srcOrientation\":\"Right\"},\"iconPlacement\":\"left\",\"opacity\":1,\"position\":[0.09603365384615385,0.46033653846153844],\"show\":true,\"text\":{\"content\":\"0\",\"font\":\"Helvetica\",\"fontSize\":24}},\"Value\":0},{\"Label\":{\"color\":[0,0,0,1],\"icon\":{\"size\":[0,0],\"src\":[],\"srcOrientation\":\"Right\"},\"iconPlacement\":\"left\",\"opacity\":1,\"position\":[0.7191706730769231,0.19501201923076922],\"show\":true,\"text\":{\"content\":\"32\",\"font\":\"Helvetica\",\"fontSize\":24}},\"Value\":32},{\"Label\":{\"color\":[0,0,0,1],\"icon\":{\"size\":[0,0],\"src\":[],\"srcOrientation\":\"Right\"},\"iconPlacement\":\"left\",\"opacity\":1,\"position\":[0.7191706730769231,0.19501201923076922],\"show\":true,\"text\":{\"content\":\"64\",\"font\":\"Helvetica\",\"fontSize\":24}},\"Value\":64},{\"Label\":{\"color\":[0,0,0,1],\"icon\":{\"size\":[0,0],\"src\":[],\"srcOrientation\":\"Right\"},\"iconPlacement\":\"left\",\"opacity\":1,\"position\":[0.7191706730769231,0.19501201923076922],\"show\":true,\"text\":{\"content\":\"96\",\"font\":\"Helvetica\",\"fontSize\":24}},\"Value\":96},{\"Label\":{\"color\":[0,0,0,1],\"icon\":{\"size\":[0,0],\"src\":[],\"srcOrientation\":\"Right\"},\"iconPlacement\":\"left\",\"opacity\":1,\"position\":[0.7191706730769231,0.19501201923076922],\"show\":true,\"text\":{\"content\":\"127\",\"font\":\"Helvetica\",\"fontSize\":24}},\"Value\":127}],\"tickRadius\":0.32}},{\"name\":\"BackgroundImageComponent\",\"settings\":{\"image\":{\"size\":[155,150],\"src\":\"data:image\\/svg+xml;base64,PD94bWwgdmVyc2lvbj0iMS4wIiBlbmNvZGluZz0idXRmLTgiPz4NCjwhLS0gR2VuZXJhdG9yOiBBZG9iZSBJbGx1c3RyYXRvciAyNS4wLjAsIFNWRyBFeHBvcnQgUGx1Zy1JbiAuIFNWRyBWZXJzaW9uOiA2LjAwIEJ1aWxkIDApICAtLT4NCjxzdmcgdmVyc2lvbj0iMS4xIg0KCSBpZD0iTGF5ZXJfMl8xXyIgeG1sbnM6Y2M9Imh0dHA6Ly9jcmVhdGl2ZWNvbW1vbnMub3JnL25zIyIgeG1sbnM6ZGM9Imh0dHA6Ly9wdXJsLm9yZy9kYy9lbGVtZW50cy8xLjEvIiB4bWxuczppbmtzY2FwZT0iaHR0cDovL3d3dy5pbmtzY2FwZS5vcmcv ...(+4184 chars)\",\"srcOrientation\":\"Right\"},\"position\":[0,0,1,1],\"scaleMode\":\"0\"}},{\"name\":\"ForegroundImageComponent\",\"settings\":{\"image\":{\"size\":[0,0],\"src\":\"default\",\"srcOrientation\":[]},\"isForeground\":1,\"position\":[0,0,1,1],\"scaleMode\":\"0\"}}],\"settings\":{\"BindingType\":\"param\",\"backgroundColor\":[0,0,255,\"1\"],\"backgroundOffset\":1,\"fixedAspectRatio\":\"on\",\"image\":{\"size\":[150,150],\"src\":\"data:image\\/svg+xml;base64,PD94bWwgdmVyc2lvbj0iMS4wIiBlbmNvZGluZz0iVVRGLTgiIHN0YW5kYWxvbmU9Im5vIj8+CjwhLS0gR2VuZXJhdG9yOiBBZG9iZSBJbGx1c3RyYXRvciAxOS4yLjEsIFNWRyBFeHBvcnQgUGx1Zy1JbiAuIFNWRyBWZXJzaW9uOiA2LjAwIEJ1aWxkIDApICAtLT4KCjxzdmcKICAgeG1sbnM6ZGM9Imh0dHA6Ly9wdXJsLm9yZy9kYy9lbGVtZW50cy8xLjEvIgogICB4bWxuczpjYz0iaHR0cDovL2NyZWF0aXZlY29tbW9ucy5vcmcvbnMjIgogICB4bWxuczpyZGY9Imh0dHA6Ly93d3cudzMub3JnLzE5OTkvMDIvMjItcmRmLXN5bnRh ...(+9660 chars)\"},\"showBackgroundColor\":false,\"variant\":\"rotarySwitch\",\"version\":\"R2022b\"},\"type\":\"RotarySwitch\"}"
